simulink model "twoFingerSim"  (R2015b)
settings: Solver=VariableStepAuto  StartTime=0.0  StopTime=1  RelTol=1e-3
settings Model: Creator=Ricardo  LastModifiedBy=Ricardo

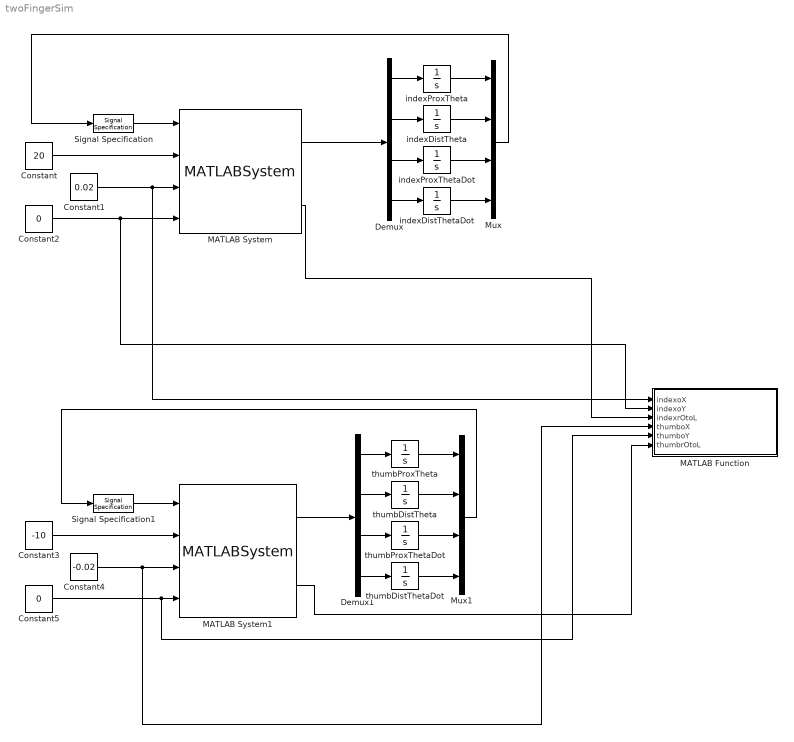
== system twoFingerSim ==
  Constant : Constant  Value=20
  Constant1 : Constant  Value=0.02
  Constant2 : Constant  Value=0
  Constant3 : Constant  Value=-10
  Constant4 : Constant  Value=-0.02
  Constant5 : Constant  Value=0
  Demux : Demux
  Demux1 : Demux
  MATLAB Function : MATLAB Function  TreatAsAtomicUnit=on
  MATLAB System : MATLABSystem  System=Index  kP=-1  kD=-5  dP=-0.01  dD=-0.01  lP=0.1  lD=0.1  rP=0.02  rD=0.012  mP=0.02  mD=0.02  thetaP=pi/10  thetaD=pi/3  SimulateUsing=Code generation
      mask Type: Index
      mask Display:
      | disp('Index');
      | port_label('input',1,'initVal');
      | port_label('input',2,'fa');
      | port_label('input',3,'oX');
      | port_label('input',4,'oY');
      | port_label('output',1,'xDot');
      | port_label('output',2,'rOtoL');
  MATLAB System1 : MATLABSystem  System=Thumb  kP=-1  kD=-5  dP=-0.01  dD=-0.01  lP=0.1  lD=0.1  rP=0.02  rD=0.012  mP=0.02  mD=0.02  thetaP=pi-pi/10  thetaD=-pi/3  SimulateUsing=Code generation
      mask Type: Thumb
      mask Display:
      | disp('Thumb');
      | port_label('input',1,'initVal');
      | port_label('input',2,'fa');
      | port_label('input',3,'oX');
      | port_label('input',4,'oY');
      | port_label('output',1,'xDot');
      | port_label('output',2,'rOtoL');
  Mux : Mux
  Mux1 : Mux
  Signal Specification : SignalSpecification  Dimensions=4
  Signal Specification1 : SignalSpecification  Dimensions=4
  indexDistTheta : Integrator  InitialCondition=pi/3  ContinuousStateAttributes='indexDistTheta'
  indexDistThetaDot : Integrator  ContinuousStateAttributes='indexDistThetaDot'
  indexProxTheta : Integrator  InitialCondition=pi/10  ContinuousStateAttributes='indexProxTheta'
  indexProxThetaDot : Integrator  ContinuousStateAttributes='indexProxThetaDot'
  thumbDistTheta : Integrator  InitialCondition=-pi/3  ContinuousStateAttributes='thumbDistTheta'
  thumbDistThetaDot : Integrator  ContinuousStateAttributes='thumbDistThetaDot'
  thumbProxTheta : Integrator  InitialCondition=pi-pi/10  ContinuousStateAttributes='thumbProxTheta'
  thumbProxThetaDot : Integrator  ContinuousStateAttributes='thumbProxThetaDot'
  wires:
  Demux/1 -> indexProxTheta/1
  Demux/2 -> indexDistTheta/1
  Demux/3 -> indexProxThetaDot/1
  Demux/4 -> indexDistThetaDot/1
  MATLAB System/1 -> Demux/1
  Constant/1 -> MATLAB System/2
  Constant1/1 -> MATLAB Function/1(indexoX), MATLAB System/3
  Constant2/1 -> MATLAB Function/2(indexoY), MATLAB System/4
  Demux1/1 -> thumbProxTheta/1
  Demux1/2 -> thumbDistTheta/1
  Demux1/3 -> thumbProxThetaDot/1
  Demux1/4 -> thumbDistThetaDot/1
  MATLAB System1/1 -> Demux1/1
  Constant3/1 -> MATLAB System1/2
  Constant4/1 -> MATLAB Function/4(thumboX), MATLAB System1/3
  Constant5/1 -> MATLAB Function/5(thumboY), MATLAB System1/4
  indexProxTheta/1 -> Mux/1
  indexDistTheta/1 -> Mux/2
  indexProxThetaDot/1 -> Mux/3
  indexDistThetaDot/1 -> Mux/4
  Mux/1 -> Signal Specification/1
  thumbProxTheta/1 -> Mux1/1
  thumbDistTheta/1 -> Mux1/2
  thumbProxThetaDot/1 -> Mux1/3
  thumbDistThetaDot/1 -> Mux1/4
  Mux1/1 -> Signal Specification1/1
  MATLAB System1/2 -> MATLAB Function/6(thumbrOtoL)
  MATLAB System/2 -> MATLAB Function/3(indexrOtoL)
  Signal Specification1/1 -> MATLAB System1/1
  Signal Specification/1 -> MATLAB System/1

== matlab function twoFingerSim/MATLAB Function ==
  data: indexoX input; indexoY input; indexrOtoL input; thumboX input; thumboY input; thumbrOtoL input
function plotSim(indexoX,indexoY,indexrOtoL,thumboX,thumboY,thumbrOtoL)
%#codegen
    % Call figure
    figure(1);
    clf;
    hold on;
    % Draw Proximal components of finger
%     viscircles(finger.origin,0.005,'Color', 'k','LineWidth',8);
    plot([indexoX indexrOtoL(1,1)],[indexoY indexrOtoL(2,1)],'LineWidth',8,'Color', 'k');
    % Draw Distal components of finger
%     viscircles(rOtoL(:,1)',0.005,'Color', 'k','LineWidth',8);
    plot([indexrOtoL(1,1) indexrOtoL(1,2)],[indexrOtoL(2,1) indexrOtoL(2,2)],'LineWidth',8,'Color', 'k');
    % Draw fingertip
%     viscircles(rOtoL(:,2)',0.003,'Color', 'k','LineWidth',8);
    plot([thumboX thumbrOtoL(1,1)],[thumboY thumbrOtoL(2,1)],'LineWidth',8,'Color', 'k');
    plot([thumbrOtoL(1,1) thumbrOtoL(1,2)],[thumbrOtoL(2,1) thumbrOtoL(2,2)],'LineWidth',8,'Color', 'k');
    hold off;
    axis([-0.2 0.2 -0.05 0.2]);
end
